simulink model "Lab3_ThyristorControlledRectifier"  (R2019a)
settings: Solver=FixedStepDiscrete  StartTime=0.0  StopTime=2  RelTol=1e-3
undefined symbols (not defined in the file): D1, lagging, pulse, R1
libraries: powerlib x24, powerlib_meascontrol x9, eePowerMeasurement x1
settings Model: Creator=ryusl  LastModifiedBy=ryusl

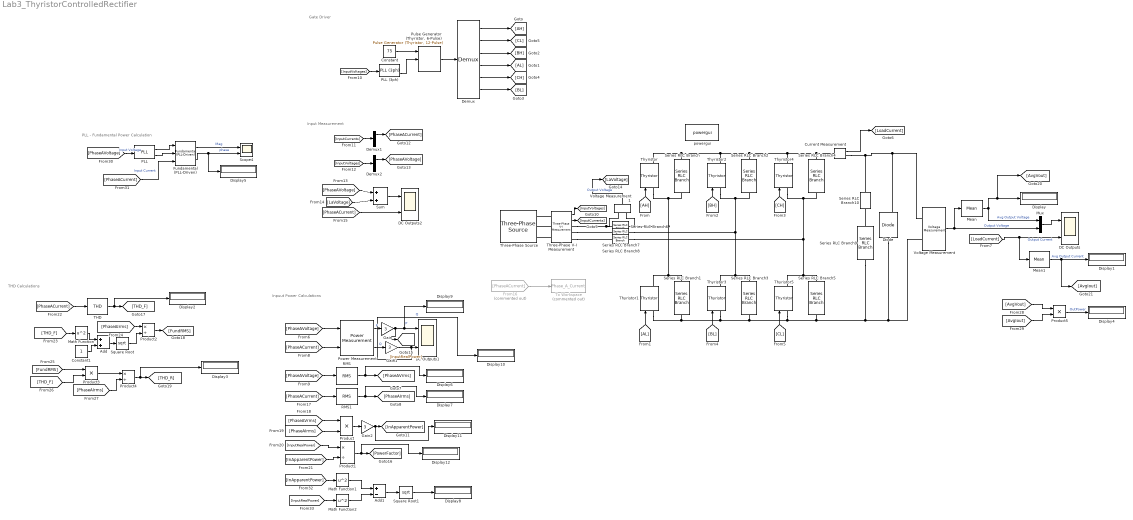
== system Lab3_ThyristorControlledRectifier ==
  note: Inpuut Power Calculations
  note: THD Calculations
  note: Input Measurement
  note: Gate Driver
  note: PLL - Fundamental Power Calculation
  Add : Sum
  Add1 : Sum  Inputs=+-
  Constant : Constant  Value=75
  Constant1 : Constant
  Current Measurement : powerlib/Measurements/Current Measurement  PhasorSimulation=off  OutputType=Complex  PSBequivalent=0
      settings: SourceProductName=Simscape Electrical
  DC Outputs : Scope  NumInputPorts=2
  DC Outputs1 : Scope  NumInputPorts=2
  DC Outputs2 : Scope  NumInputPorts=2
  Demux : Demux  Outputs=6
  Demux1 : Demux  Outputs=3
  Demux2 : Demux  Outputs=3
  Diode : powerlib/Power Electronics/Diode  Ron=0.001  Lon=0  Vf=0.001  IC=0  UseSnubber=0  Rs=0  Cs=0  Measurements=on
      settings: SourceProductName=Simscape Electrical
  Display{,1..12} (13 alike) : Display
  From16 : From  Commented=on  GotoTag=PhaseACurrent
  Fundamental (PLL-Driven) : powerlib_meascontrol/Measurements/Fundamental (PLL-Driven)  Finit=50  Fmin=50  InInit=[1, 0]  Ts=1e-5
      settings: SourceProductName=Simscape Electrical  SourceProductBaseCode=PS
  Gain : Gain  Gain=3
  Gain1 : Gain  Gain=3
  Gain2 : Gain  Gain=3
  Math Function : Math  Operator=square  SaturateOnIntegerOverflow=on
  Math Function1 : Math  Operator=square  SaturateOnIntegerOverflow=on
  Math Function2 : Math  Operator=square  SaturateOnIntegerOverflow=on
  Mean : powerlib_meascontrol/Measurements/Mean  Freq=300  Vinit=0  Ts=1e-5
      settings: SourceProductName=Simscape Electrical
  Mean1 : powerlib_meascontrol/Measurements/Mean  Freq=300  Vinit=0  Ts=1e-6
      settings: SourceProductName=Simscape Electrical
  Mux : Mux  Inputs=2
  PLL : powerlib_meascontrol/PLL/PLL  Fmin=45  Par_Init=[0, 60]  ParK=[180, 3200, 1]  TcD=1e-4  MaxRateChangeFreq=12  FilterCutOffFreq=25  Ts=1e-5  AGC=on
      settings: SourceProductName=Simscape Electrical  SourceProductBaseCode=PS
  PLL (3ph) : powerlib_meascontrol/PLL/PLL (3ph)  Fmin=45  Par_Init=[0, 60]  ParK=[180, 3200, 1]  TcD=1e-4  MaxRateChangeFreq=12  FilterCutOffFreq=25  Ts=10e-5  AGC=on
      settings: SourceProductName=Simscape Electrical
  Power Measurement : eePowerMeasurement/Power Measurement  LabelModeActiveChoice=Discrete  F=50  K=[1]  Ts=1e-5
      settings: SourceProductName=Simscape Electrical  SourceProductBaseCode=PS
  Product : Product
  Product1 : Product  Inputs=*/
  Product2 : Product  Inputs=*/
  Product3 : Product
  Product4 : Product  Inputs=*/
  Product5 : Product
  "Pulse Generator (Thyristor, 6-Pulse)" : powerlib_meascontrol/Pulse & Signal Generators/Pulse Generator (Thyristor, 12-Pulse)  GenType=6-pulse  Delta=D1 (lagging)  pwidth=60  Double_Pulse=off  Ts=10e-5
      settings: SourceProductName=Simscape Electrical  SourceProductBaseCode=PS
  RMS : powerlib_meascontrol/Measurements/RMS  TrueRMS=off  Freq=50  RMSInit=0  Ts=1e-5
      settings: SourceProductName=Simscape Electrical
  RMS1 : powerlib_meascontrol/Measurements/RMS  TrueRMS=off  Freq=50  RMSInit=0  Ts=1e-5
      settings: SourceProductName=Simscape Electrical
  Scope4 : Scope  NumInputPorts=2
  Series RLC Branch{,1..5} (6 alike) : powerlib/Elements/Series RLC Branch  LConnTagsString=__new0  RConnTagsString=__new0  BranchType=R  Resistance=1e6  Inductance=1e-3  SetiL0=off  InitialCurrent=0  Capacitance=1e-6  Setx0=off  InitialVoltage=0  Measurements=None
      settings: SourceProductName=Simscape Electrical
  Series RLC Branch10 : powerlib/Elements/Series RLC Branch  LConnTagsString=__new0  RConnTagsString=__new0  BranchType=L  Resistance=1e6  Inductance=0.4575  SetiL0=off  InitialCurrent=0  Capacitance=1e-6  Setx0=off  InitialVoltage=0  Measurements=None
      settings: SourceProductName=Simscape Electrical
  Series RLC Branch6 : powerlib/Elements/Series RLC Branch  LConnTagsString=__new0  RConnTagsString=__new0  BranchType=L  Resistance=1e6  Inductance=5e-3  SetiL0=off  InitialCurrent=0  Capacitance=1e-6  Setx0=off  InitialVoltage=0  Measurements=None
      settings: SourceProductName=Simscape Electrical
  Series RLC Branch7 : powerlib/Elements/Series RLC Branch  LConnTagsString=__new0  RConnTagsString=__new0  BranchType=L  Resistance=1e6  Inductance=5e-3  SetiL0=off  InitialCurrent=0  Capacitance=1e-6  Setx0=off  InitialVoltage=0  Measurements=None
      settings: SourceProductName=Simscape Electrical
  Series RLC Branch8 : powerlib/Elements/Series RLC Branch  LConnTagsString=__new0  RConnTagsString=__new0  BranchType=L  Resistance=1e6  Inductance=5e-3  SetiL0=off  InitialCurrent=0  Capacitance=1e-6  Setx0=off  InitialVoltage=0  Measurements=None
      settings: SourceProductName=Simscape Electrical
  Series RLC Branch9 : powerlib/Elements/Series RLC Branch  LConnTagsString=__new0  RConnTagsString=__new0  BranchType=R  Resistance=(3*R1)/8  Inductance=1e-3  SetiL0=off  InitialCurrent=0  Capacitance=1e-6  Setx0=off  InitialVoltage=0  Measurements=None
      settings: SourceProductName=Simscape Electrical
  Square Root : Sqrt  SaturateOnIntegerOverflow=on
  Square Root1 : Sqrt  SaturateOnIntegerOverflow=on
  Sum : Sum  Inputs=+|+
  THD : powerlib_meascontrol/Measurements/THD  Freq=50  Ts=1e-5
      settings: SourceProductName=Simscape Electrical
  Three-Phase V-I Measurement : powerlib/Measurements/Three-Phase V-I Measurement  VoltageMeasurement=phase-to-ground  SetLabelV=off  LabelV=Vabc  Vpu=off  VpuLL=off  CurrentMeasurement=yes  SetLabelI=off  LabelI=Iabc  Ipu=off  Pbase=100e6  Vbase=500e3  OutputType=Complex  PhasorSimulation=off  PSBequivalent=0
      settings: SourceProductName=Simscape Electrical
  Three-Phase Source : powerlib/Electrical Sources/Three-Phase Source  InternalConnection=Yg  VoltagePhases=off  Voltage=200*sqrt(3/2)  PhaseAngle=0  Voltage_phases=[25e3 25e3 25e3]/sqrt(3)  PhaseAngles_phases=[0 -120 +120]  Frequency=50  NonIdealSource=off  SpecifyImpedance=off  Resistance=0  Inductance=0  ShortCircuitLevel=100e6  BaseVoltage=0  XRratio=7  BusType=swing  Pref=10e3  Qref=0  Prefabc=[10e3, 10e3, 10e3]  Qrefabc=[0, 0, 0]  Qmin=-inf  Qmax=inf
      settings: SourceProductName=Simscape Electrical
  Thyristor{,1..5} (6 alike) : powerlib/Power Electronics/Thyristor  Ron=1e-6  Lon=0  Vf=1e-8  IC=0  Rs=0  Cs=0  Measurements=on
      settings: SourceProductName=Simscape Electrical
  To Workspace : ToWorkspace  Commented=on  VariableName=Phase_A_Current  SaveFormat=Structure With Time  SampleTime=-1
  Voltage Measurement : powerlib/Measurements/Voltage Measurement  PhasorSimulation=off  OutputType=Complex  PSBequivalent=0
      settings: SourceProductName=Simscape Electrical
  Voltage Measurement1 : powerlib/Measurements/Voltage Measurement  PhasorSimulation=off  OutputType=Complex  PSBequivalent=0
      settings: SourceProductName=Simscape Electrical
  powergui : powerlib/powergui  Priority=1  SimulationMode=Discrete  SampleTime=5e-6  frequency=60  Iterations=50  frequencyindice=0  Pbase=100e6  ErrMax=1e-4  UnitsV=kV  UnitsW=MW  buscounter=0  FunctionMessages=off  echomessages=off  EnableUseOfTLC=off  CurrentSourceSwitches=off  DisableSnubberDevices=off  DisableRonSwitches=off  DisableVfSwitches=off  DisplayEquations=off  AutomaticDiscreteSolvers=off  SolverType=Tustin/Backward Euler (TBE)  Interpol=off  ExternalGateDelay=off  methode=off  Ts=100  x0status=blocks  SPID=on  SwTol=0  HookPort=off  NonlinearTolerance=0  nMaxIteration=15  ContinueOnMaxIteration=off  RestoreLinks=warning  ResistiveCurrentMeasurement=off  Frange=[0:2:500]  Ylog=off  Xlog=on  ShowGrid=off  save=off  variable=ZData  structure=Phase_A_Current  ZoomFFT=off  StartTime=0.8  cycles=5  DisplayStyle=1  fundamental=50  FreqAxis=on  MaxFrequency=1000  frequencyindicesteady=1  RmsSteady=1  display=off
      settings: SourceProductName=Simscape Electrical
  wires:
  Demux/2 -> [CL]
  Current Measurement/1 -> [LoadCurrent]
  Demux/5 -> [CH]
  Demux/1 -> [AH]
  Voltage Measurement/1 -> Mean/1, Mux/2  "Output Voltage"
  [BH] -> Thyristor2/1
  Demux/6 -> [BL]
  Demux/3 -> [BH]
  Constant/1 -> "Pulse Generator (Thyristor, 6-Pulse)"/1
  [CL] -> Thyristor5/1
  [AL] -> Thyristor1/1
  [AH] -> Thyristor/1
  [CH] -> Thyristor4/1
  Demux2/1 -> [PhaseAVoltage]
  Sum/1 -> DC Outputs2/1
  [BL] -> Thyristor3/1
  [InputCurrents] -> Demux1/1
  PLL (3ph)/2 -> "Pulse Generator (Thyristor, 6-Pulse)"/2
  Mux/1 -> DC Outputs/1
  From16/1 -> To Workspace/1
  "Pulse Generator (Thyristor, 6-Pulse)"/1 -> Demux/1
  [PhaseAVoltage] -> Sum/1
  [LoadCurrent] -> Mean1/1, DC Outputs/2  "Output Current"
  Mean1/1 -> [AvgIout], Display1/1  "Avg Output Current"
  [LaVoltage] -> Sum/2
  [PhaseACurrent] -> DC Outputs2/2
  Demux1/1 -> [PhaseACurrent]
  Voltage Measurement1/1 -> [LaVoltage]  "Output Voltage"
  Three-Phase V-I Measurement/2 -> [InputCurrents]
  Demux/4 -> [AL]
  [InputVoltages] -> PLL (3ph)/1
  Mean/1 -> Mux/1, [AvgVout], Display/1  "Avg Output Voltage"
  [InputVoltages] -> Demux2/1
  Three-Phase V-I Measurement/1 -> [InputVoltages]
  [PhaseAVoltage] -> Power Measurement/1
  [PhaseACurrent] -> Power Measurement/2
  [PhaseAVoltage] -> RMS/1
  [PhaseACurrent] -> RMS1/1
  RMS/1 -> Display6/1, [PhaseAVrms]
  RMS1/1 -> Display7/1, [PhaseAIrms]
  [PhaseAVrms] -> Product/1
  [PhaseAIrms] -> Product/2
  Product/1 -> Gain2/1
  [InputRealPower] -> Product1/1
  [InApparentPower] -> Product1/2
  Product1/1 -> Display12/1, [PowerFactor]
  [PhaseACurrent] -> THD/1
  THD/1 -> Display2/1, [THD_F]
  [THD_F] -> Math Function/1
  Math Function/1 -> Add/1
  Constant1/1 -> Add/2
  Add/1 -> Square Root/1
  Square Root/1 -> Product2/2
  [PhaseAIrms] -> Product2/1
  Product2/1 -> [FundRMS]
  [FundRMS] -> Product3/1
  [THD_F] -> Product3/2
  Product3/1 -> Product4/1
  [PhaseAIrms] -> Product4/2
  Product4/1 -> Display3/1, [THD_R]
  [AvgVout] -> Product5/1
  [AvgIout] -> Product5/2
  Product5/1 -> Display4/1  "OutPower"
  PLL/2 -> Fundamental (PLL-Driven)/2
  [PhaseAVoltage] -> PLL/1  "Input Voltage"
  PLL/1 -> Fundamental (PLL-Driven)/1
  Fundamental (PLL-Driven)/2 -> Display5/1, Scope4/2  "phase"
  [PhaseACurrent] -> Fundamental (PLL-Driven)/3  "Input Current"
  Fundamental (PLL-Driven)/1 -> Scope4/1  "Mag"
  [InApparentPower] -> Math Function1/1
  [InputRealPower] -> Math Function2/1
  Math Function1/1 -> Add1/1
  Math Function2/1 -> Add1/2
  Add1/1 -> Square Root1/1
  Square Root1/1 -> Display8/1
  Gain/1 -> DC Outputs1/1, Display9/1, [InputRealPower]  "P"
  Gain2/1 -> Display11/1, [InApparentPower]
  Power Measurement/1 -> Gain/1  "P"
  Power Measurement/2 -> Gain1/1  "Q"
  Gain1/1 -> Display10/1, DC Outputs1/2  "Q"
  connections:
  Thyristor5/RConn1 -- Series RLC Branch5/LConn1 -- Series RLC Branch8/LConn1 -- Thyristor4/LConn1 -- Series RLC Branch4/RConn1
  Current Measurement/RConn1 -- Series RLC Branch10/RConn1 -- Diode/RConn1 -- Voltage Measurement/LConn1
  Voltage Measurement/LConn2 -- Diode/LConn1 -- Series RLC Branch9/RConn1 -- Thyristor1/LConn1 -- Series RLC Branch1/RConn1 -- Thyristor3/LConn1 -- Series RLC Branch3/RConn1 -- Thyristor5/LConn1 -- Series RLC Branch5/RConn1
  Thyristor/LConn1 -- Series RLC Branch6/LConn1 -- Voltage Measurement1/LConn2 -- Series RLC Branch1/LConn1 -- Thyristor1/RConn1 -- Series RLC Branch/RConn1
  Series RLC Branch3/LConn1 -- Thyristor3/RConn1 -- Series RLC Branch7/LConn1 -- Thyristor2/LConn1 -- Series RLC Branch2/RConn1
  Series RLC Branch/LConn1 -- Thyristor/RConn1 -- Current Measurement/LConn1 -- Series RLC Branch4/LConn1 -- Thyristor4/RConn1 -- Series RLC Branch2/LConn1 -- Thyristor2/RConn1
  Three-Phase V-I Measurement/LConn3 -- Three-Phase Source/RConn3
  Three-Phase V-I Measurement/LConn2 -- Three-Phase Source/RConn2
  Three-Phase V-I Measurement/LConn1 -- Three-Phase Source/RConn1
  Series RLC Branch9/LConn1 -- Series RLC Branch10/LConn1
  Three-Phase V-I Measurement/RConn3 -- Series RLC Branch8/RConn1
  Three-Phase V-I Measurement/RConn2 -- Series RLC Branch7/RConn1
  Three-Phase V-I Measurement/RConn1 -- Voltage Measurement1/LConn1 -- Series RLC Branch6/RConn1
